simulink model "DeMux_Sensor_Data"  (R2021a)
settings: Solver=VariableStepAuto  StartTime=0.0  StopTime=10.0  RelTol=1e-3
settings Model: Creator=mojta  LastModifiedBy=mojta

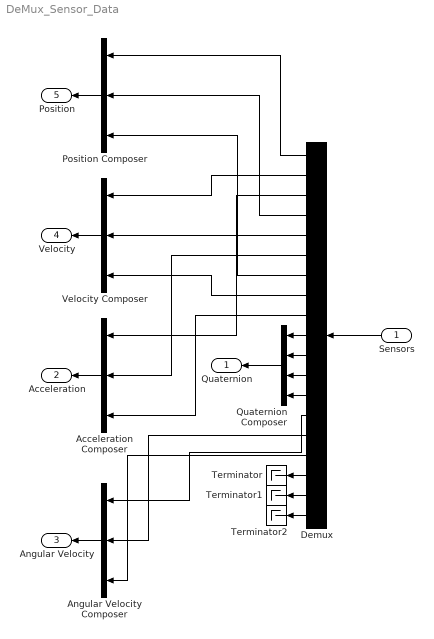
== system DeMux_Sensor_Data ==
  Sensors : Inport
  Acceleration Composer : Mux  Inputs=3
  Angular Velocity Composer : Mux  Inputs=3
  Demux : Demux  Outputs=9+4+3+3
  Position Composer : Mux  Inputs=3
  Quaternion Composer : Mux
  Terminator : Terminator
  Terminator1 : Terminator
  Terminator2 : Terminator
  Velocity Composer : Mux  Inputs=3
  Quaternion : Outport
  Acceleration : Outport  Port=2
  Angular Velocity : Outport  Port=3
  Velocity : Outport  Port=4
  Position : Outport  Port=5
  wires:
  Sensors/1 -> Demux/1
  Demux/1 -> Position Composer/1
  Demux/4 -> Position Composer/2
  Demux/7 -> Position Composer/3
  Demux/2 -> Velocity Composer/1
  Demux/5 -> Velocity Composer/2
  Demux/8 -> Velocity Composer/3
  Demux/3 -> Acceleration Composer/1
  Demux/6 -> Acceleration Composer/2
  Demux/9 -> Acceleration Composer/3
  Demux/16 -> Angular Velocity Composer/3
  Demux/15 -> Angular Velocity Composer/2
  Demux/14 -> Angular Velocity Composer/1
  Demux/10 -> Quaternion Composer/1
  Demux/11 -> Quaternion Composer/2
  Demux/12 -> Quaternion Composer/3
  Demux/13 -> Quaternion Composer/4
  Quaternion Composer/1 -> Quaternion/1
  Acceleration Composer/1 -> Acceleration/1
  Angular Velocity Composer/1 -> Angular Velocity/1
  Velocity Composer/1 -> Velocity/1
  Position Composer/1 -> Position/1
  Demux/17 -> Terminator/1
  Demux/18 -> Terminator1/1
  Demux/19 -> Terminator2/1
